simulink model "practice1"  (R2014a)
settings: Solver=ode45  StartTime=0.0  StopTime=10.0  RelTol=1e-3
settings Model: Creator=Huanglei  LastModifiedBy=Huanglei

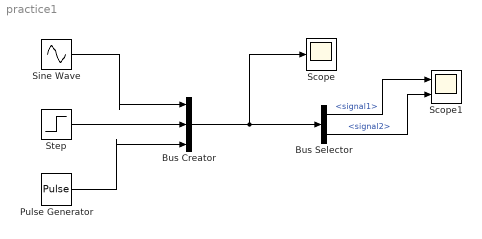
== system practice1 ==
  Bus Creator : BusCreator  Inputs=3
  Bus Selector : BusSelector  OutputSignals=signal1,signal2
  Pulse Generator : DiscretePulseGenerator  PulseType=Time based  Period=0.1  PulseWidth=5
  Scope : Scope
  Scope1 : Scope  NumInputPorts=2
      settings: YMin=-5~-5  YMax=5~5
  Sine Wave : Sin  SampleTime=0
  Step : Step  Time=1.5  After=0.5  SampleTime=0
  wires:
  Step/1 -> Bus Creator/2
  Pulse Generator/1 -> Bus Creator/3
  Sine Wave/1 -> Bus Creator/1
  Bus Creator/1 -> Scope/1, Bus Selector/1
  Bus Selector/1 -> Scope1/1  "<signal1>"
  Bus Selector/2 -> Scope1/2  "<signal2>"
